simulink model "adaptiveexactgain"  (Simulink 7.5)
settings: Solver=ode45  StartTime=0.0  StopTime=10.0  RelTol=1e-3
InitFcn:
  | startup_exact
values from neighbouring files (symbols this model uses):
  am = 5    [startup_adaptive.m]    (also in startup_exact.m)
  f1 = 5.0991    [startup_adaptive.m]    (also in startup_exact.m)
  f2 = 85.3455    [startup_adaptive.m]    (also in startup_exact.m)
  g1 = 13.8    [startup_adaptive.m]    (also in startup_exact.m)
  g2 = 41.1089    [startup_adaptive.m]    (also in startup_exact.m)
  kr = -45.4545    [startup_exact.m]
  T = [1 2*zeta*wn wn^2]    [startup_adaptive.m]    (also in startup_exact.m)
libraries: simulink x2
settings Model: Creator=Prasad  LastModifiedBy=Prasad

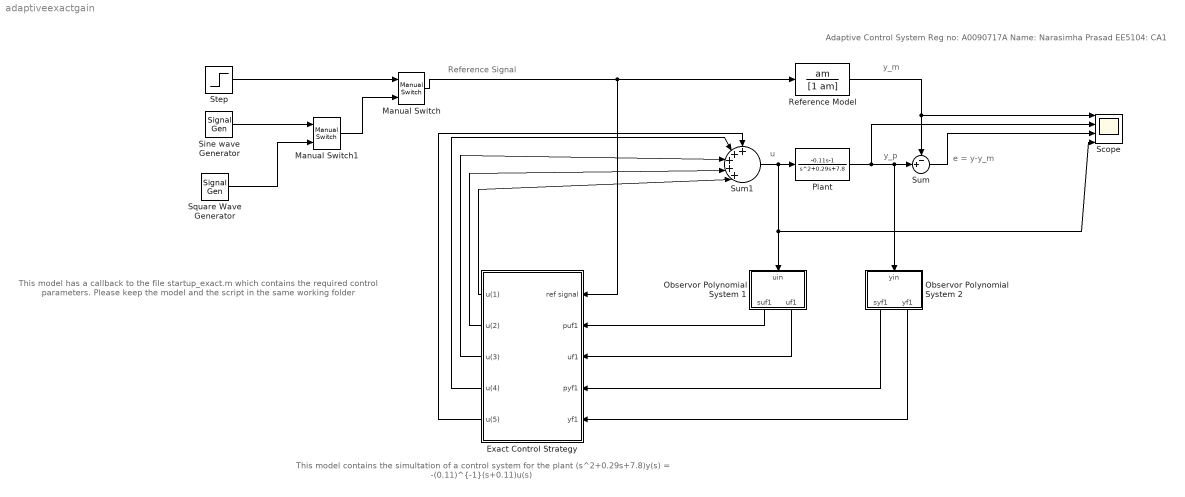
== system adaptiveexactgain ==
  note: Adaptive Control System
      | Reg no: A0090717A
      | Name: Narasimha Prasad
      | EE5104: CA1
  note: This model has a callback
      | to the file startup_exact.m which
      | contains the required control
      | parameters. Please keep
      |  the model and the script
      | in the same working folder
  note: Reference Signal
  note: u
  note: y_p
  note: y_m
  note: e = y-y_m
  note: This model contains the simultation of a control system for the plant (s^2+0.29s+7.8)y(s) = -(0.11)^{-1}(s+0.11)u(s)
  Exact Control Strategy : Subsystem
  Manual Switch : simulink/Signal Routing/Manual Switch  SystemSampleTime=-1  sw=1  action=0  varsize=off
  Manual Switch1 : simulink/Signal Routing/Manual Switch  SystemSampleTime=-1  sw=1  action=0  varsize=off
  Observor Polynomial System 1 : Subsystem
  Observor Polynomial System 2 : Subsystem
  Plant : TransferFcn  Numerator=[-0.11 -1]  Denominator=[1 0.29 7.8]
  Reference Model : TransferFcn  Numerator=am  Denominator=[1 am]
  Scope : Scope  NumInputPorts=4
      settings: TimeRange=20  YMin=0~-5~-5~-5  YMax=1.5~5~5~5
  Sine wave Generator : SignalGenerator  Amplitude=10  Frequency=2  Units=rad/sec
  Square Wave Generator : SignalGenerator  WaveForm=square  Frequency=2.2  Units=rad/sec
  Step : Step  SampleTime=0
  Sum : Sum  Inputs=-+|  OutDataType=fixdt(1, 16)  OutScaling=2^0
  Sum1 : Sum  Inputs=+++++|  OutDataType=fixdt(1, 16)  OutScaling=2^0
  wires:
  Reference Model/1 -> Sum/1, Scope/1
  Plant/1 -> Sum/2, Observor Polynomial System 2/1(yin), Scope/2
  Sum1/1 -> Plant/1, Observor Polynomial System 1/1(uin), Scope/4
  Sum/1 -> Scope/3
  Manual Switch/1 -> Reference Model/1, Exact Control Strategy/1(ref signal)
  Sine wave Generator/1 -> Manual Switch1/1
  Square Wave Generator/1 -> Manual Switch1/2
  Step/1 -> Manual Switch/1
  Manual Switch1/1 -> Manual Switch/2
  Exact Control Strategy/1(u(1)) -> Sum1/5
  Exact Control Strategy/2(u(2)) -> Sum1/4
  Exact Control Strategy/3(u(3)) -> Sum1/3
  Exact Control Strategy/4(u(4)) -> Sum1/2
  Exact Control Strategy/5(u(5)) -> Sum1/1
  Observor Polynomial System 1/1(suf1) -> Exact Control Strategy/2(puf1)
  Observor Polynomial System 1/2(uf1) -> Exact Control Strategy/3(uf1)
  Observor Polynomial System 2/1(syf1) -> Exact Control Strategy/4(pyf1)
  Observor Polynomial System 2/2(yf1) -> Exact Control Strategy/5(yf1)

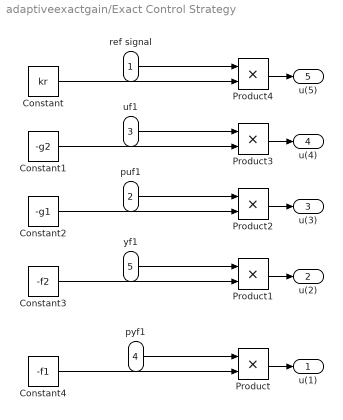
== system adaptiveexactgain/Exact Control Strategy ==
  ref signal : Inport
  puf1 : Inport  Port=2
  uf1 : Inport  Port=3
  pyf1 : Inport  Port=4
  yf1 : Inport  Port=5
  Constant : Constant  Value=kr  OutDataType=fixdt(1, 16)  OutScaling=2^0
  Constant1 : Constant  Value=-g2  OutDataType=fixdt(1, 16)  OutScaling=2^0
  Constant2 : Constant  Value=-g1  OutDataType=fixdt(1, 16)  OutScaling=2^0
  Constant3 : Constant  Value=-f2  OutDataType=fixdt(1, 16)  OutScaling=2^0
  Constant4 : Constant  Value=-f1  OutDataType=fixdt(1, 16)  OutScaling=2^0
  Product{,1..4} (5 alike) : Product  OutDataType=fixdt(1, 16)  OutScaling=2^0  RndMeth=Zero
  u(1) : Outport
  u(2) : Outport  Port=2
  u(3) : Outport  Port=3
  u(4) : Outport  Port=4
  u(5) : Outport  Port=5
  wires:
  puf1/1 -> Product2/1
  yf1/1 -> Product1/1
  pyf1/1 -> Product/1
  ref signal/1 -> Product4/1
  Product4/1 -> u(5)/1
  Product3/1 -> u(4)/1
  Product2/1 -> u(3)/1
  Product1/1 -> u(2)/1
  Product/1 -> u(1)/1
  uf1/1 -> Product3/1
  Constant/1 -> Product4/2
  Constant4/1 -> Product/2
  Constant3/1 -> Product1/2
  Constant2/1 -> Product2/2
  Constant1/1 -> Product3/2

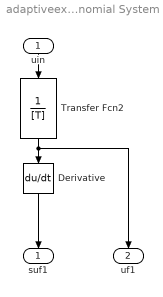
== system adaptiveexactgain/Observor Polynomial System 1 ==
  uin : Inport
  Derivative : Derivative
  Transfer Fcn2 : TransferFcn  Denominator=[T]
  suf1 : Outport
  uf1 : Outport  Port=2
  wires:
  Transfer Fcn2/1 -> uf1/1, Derivative/1
  uin/1 -> Transfer Fcn2/1
  Derivative/1 -> suf1/1

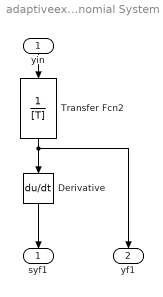
== system adaptiveexactgain/Observor Polynomial System 2 ==
  yin : Inport
  Derivative : Derivative
  Transfer Fcn2 : TransferFcn  Denominator=[T]
  syf1 : Outport
  yf1 : Outport  Port=2
  wires:
  Transfer Fcn2/1 -> yf1/1, Derivative/1
  yin/1 -> Transfer Fcn2/1
  Derivative/1 -> syf1/1
